simulink model "lin"  (Simulink 7.2)
settings: Solver=ode45  StartTime=0  StopTime=0.2
libraries: simulink x2
settings Model: Creator=Admin  LastModifiedBy=Admin
settings OptimizationCC: BooleanDataType=off  InitFltsAndDblsToZero=on
settings DebuggingCC: SaveWithParameterizedLinksMsg=none  SignalResolutionControl=TryResolveAllWithWarning  SolverPrmCheckMsg=none  MultiTaskDSMMsg=warning  MultiTaskCondExecSysMsg=none  StrictBusMsg=None
settings HardwareCC: TargetUnknown=on
settings RTWCC: IncludeERTFirstTime=on
settings GRTTargetCC: TargetFcnLib=ansi_tfl_tmw.mat

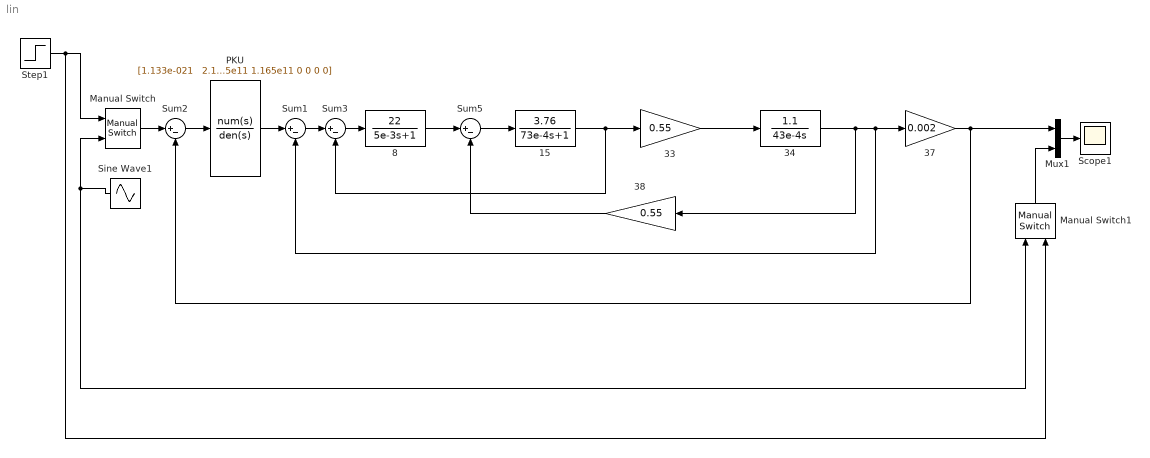
== system lin ==
  15 : TransferFcn  Numerator=[3.76]  Denominator=[73e-4 1]
  33 : Gain  Gain=0.55  ParameterDataType=sfix(16)  ParameterScaling=2^0  OutDataType=sfix(16)  OutScaling=2^0
  34 : TransferFcn  Numerator=[1.1]  Denominator=[43e-4 0]
  37 : Gain  Gain=0.002  ParameterDataType=sfix(16)  ParameterScaling=2^0  OutDataType=sfix(16)  OutScaling=2^0
  38 : Gain  Orientation=left  Gain=0.55  ParameterDataType=sfix(16)  ParameterScaling=2^0  OutDataType=sfix(16)  OutScaling=2^0
  8 : TransferFcn  Numerator=[22]  Denominator=[5e-3 1]
  Manual Switch : simulink/Signal Routing/Manual Switch  SystemSampleTime=-1  sw=0  action=0  varsize=off
  Manual Switch1 : simulink/Signal Routing/Manual Switch  Orientation=up  SystemSampleTime=-1  sw=1  action=0  varsize=off
  Mux1 : Mux  Inputs=2
  PKU : TransferFcn  Numerator="[1.133e-021   2.149e-018   7.179e-015   9.662e-12   1.32e-8   1.178e-5   0.006738 2.695 797.4 1.793e5 3.092e7 4.05e9 3.931e11 2.655e13 1.118e15 2.286e16 6.608e16 0 0 0 0]"  Denominator=[1.375e-40 2.581e-35 1.542e-30 3.734e-26 3.926e-22 1.734e-18 2.989e-15 5.009e-12 4.374e-9 2.316e-6 0.00084 0.2265 45.5 6878 7.666e5 5.962e7 2.89e9 6.806e10 2.35e11 1.165e11 0 0 0 0]
  Scope1 : Scope
      settings: TickLabels=on  TimeRange=0.1
  Sine Wave1 : Sin  Orientation=left  Frequency=200  SampleTime=0
  Step1 : Step  Time=0  SampleTime=0
  Sum{1..3,5} (4 alike) : Sum  Inputs=|+-  OutDataType=sfix(16)  OutScaling=2^0
  wires:
  Step1/1 -> Manual Switch/1, Manual Switch1/2
  Sine Wave1/1 -> Manual Switch/2, Manual Switch1/1
  8/1 -> Sum5/1
  Sum5/1 -> 15/1
  15/1 -> 33/1, Sum3/2
  33/1 -> 34/1
  34/1 -> 38/1, 37/1, Sum1/2
  38/1 -> Sum5/2
  Mux1/1 -> Scope1/1
  37/1 -> Mux1/1, Sum2/2
  Manual Switch1/1 -> Mux1/2
  Manual Switch/1 -> Sum2/1
  Sum1/1 -> Sum3/1
  Sum3/1 -> 8/1
  Sum2/1 -> PKU/1
  PKU/1 -> Sum1/1
